simulink model "s2dot3_49filter_not_good"  (R2023b)
settings: Solver=VariableStepAuto  StartTime=0.0  StopTime=10.0  RelTol=1e-3
settings Model: Creator=lxj  LastModifiedBy=lxj

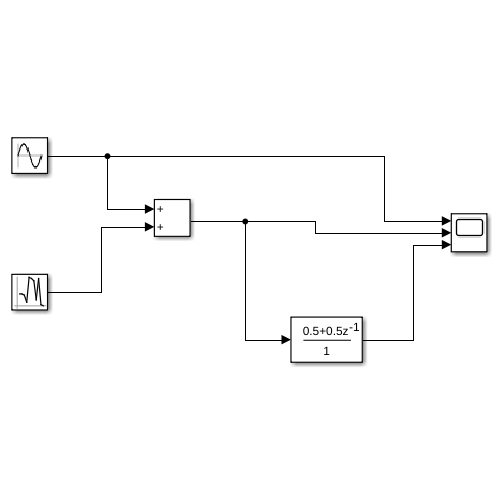
[thumbnail: Simulink's stored preview of the top-level diagram]
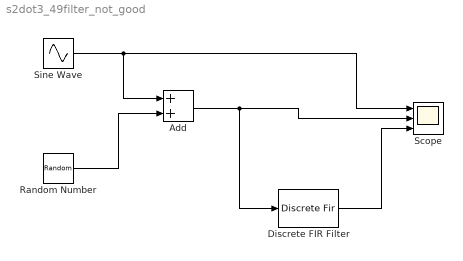
== system s2dot3_49filter_not_good ==
  Add : Sum
  Discrete FIR Filter : DiscreteFir
  Random Number : RandomNumber  Variance=0.1  SampleTime=0.1
  Scope : Scope  NumInputPorts=3
  Sine Wave : Sin  Amplitude=5  SampleTime=0
  wires:
  Sine Wave/1 -> Add/1, Scope/1
  Random Number/1 -> Add/2
  Add/1 -> Discrete FIR Filter/1, Scope/2
  Discrete FIR Filter/1 -> Scope/3
